simulink model "BLDCMotor"  (R2020a)
settings: Solver=VariableStepAuto  StartTime=0.0  StopTime=10.0  RelTol=1e-3
libraries: simulink x1
settings Model: Creator=Hp  LastModifiedBy=Hp

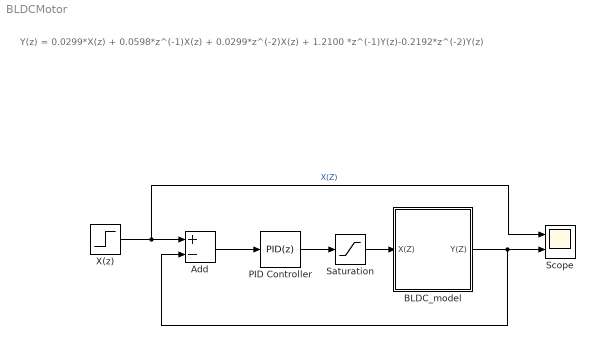
== system BLDCMotor ==
  note: Y(z) = 0.0299*X(z) + 0.0598*z^(-1)X(z) + 0.0299*z^(-2)X(z) + 1.2100 *z^(-1)Y(z)-0.2192*z^(-2)Y(z)
  Add : Sum  Inputs=+-
  BLDC_model : Subsystem
  PID Controller : simulink/Continuous/PID Controller  Controller=PID  Form=Parallel  TimeDomain=Discrete-time  UseExternalTs=off  SampleTime=-1  IntegratorMethod=Forward Euler  FilterMethod=Forward Euler  ControllerParametersSource=internal  P=1.20691388645035  I=59.4220416550733  D=0.00191645853146201  UseFilter=on  N=221.630484004673  TunerSelectOption=Transfer Function Based (PID Tuner App)  InitialConditionSource=internal  InitialConditionForIntegrator=0  InitialConditionForFilter=0  DifferentiatorICPrevScaledInput=0  ExternalReset=none  TrackingMode=off  Kt=1  LimitOutput=off  UpperSaturationLimit=inf  LowerSaturationLimit=-inf  LinearizeAsGain=on  AntiWindupMode=none  Kb=1  POutMin=[]  POutMax=[]  IOutMin=[]  IOutMax=[]  DOutMin=[]  DOutMax=[]  NOutMin=[]  NOutMax=[]  SumOutMin=[]  SumOutMax=[]  SaturationOutMin=[]  SaturationOutMax=[]  PParamMin=[]  PParamMax=[]  IParamMin=[]  IParamMax=[]  DParamMin=[]  DParamMax=[]  NParamMin=[]  NParamMax=[]  KbParamMin=[]  KbParamMax=[]  KtParamMin=[]  KtParamMax=[]  KbOutMin=[]  KbOutMax=[]  KtOutMin=[]  KtOutMax=[]  IntegratorOutMin=[]  IntegratorOutMax=[]  FilterOutMin=[]  FilterOutMax=[]  SumI1OutMin=[]  SumI1OutMax=[]  SumI2OutMin=[]  SumI2OutMax=[]  SumI3OutMin=[]  SumI3OutMax=[]  SumI4OutMin=[]  SumI4OutMax=[]  SumDOutMin=[]  SumDOutMax=[]  DifferentiatorOutMin=[]  DifferentiatorOutMax=[]  FilterDiffOutCoefMin=[]  FilterDiffOutCoefMax=[]  ReciprocalOutMin=[]  ReciprocalOutMax=[]  SumDenOutMin=[]  SumDenOutMax=[]  SumNumOutMin=[]  SumNumOutMax=[]  DivideOutMin=[]  DivideOutMax=[]  UdiffTsProdOutMin=[]  UdiffTsProdOutMax=[]  NTsProdOutMin=[]  NTsProdOutMax=[]  UintegralTsProdOutMin=[]  UintegralTsProdOutMax=[]  UngainTsProdOutMin=[]  UngainTsProdOutMax=[]  IntegratorContinuousStateAttributes=''  IntegratorStateMustResolveToSignalObject=off  IntegratorRTWStateStorageClass=Auto  FilterContinuousStateAttributes=''  FilterStateMustResolveToSignalObject=off  FilterRTWStateStorageClass=Auto  ParallelPVariant=InternalParameters  IdealPVariant=Disabled  IVariant=InternalParameters  DVariant=InternalParameters  IntegratorVariant=Discrete  SatVariant=Disabled  AWVariant=Passthrough  PCopyVariant=Disabled  TRVariant=Disabled  FdbkBlocksVariant=Forward  IdealPFdbkVariant=Disabled  SatFdbkVariant=Disabled  DerivativeFilterVariant=ForwardEulerFilter  NVariant=InternalParameters  NCopyVariant=Disabled  FilterICVariant=InternalICsFilter  IntegratorICVariant=InternalICs  ExternalResetVariant=Disabled  TRSumVariant=Passthrough  SumFdbkVariant=Disabled  SumVariant=Sum_PID  TsampFilterVariant=InternalTs  TsampNgainVariant=Passthrough  TsampIntegralVariant=Passthrough
  Saturation : Saturate  UpperLimit=1  LowerLimit=-1
  Scope : Scope  NumInputPorts=2
  X(z) : Step  SampleTime=0.001
  wires:
  X(z)/1 -> Add/1, Scope/1  "X(Z)"
  BLDC_model/1(Y(Z)) -> Add/2, Scope/2
  PID Controller/1 -> Saturation/1
  Add/1 -> PID Controller/1
  Saturation/1 -> BLDC_model/1(X(Z))

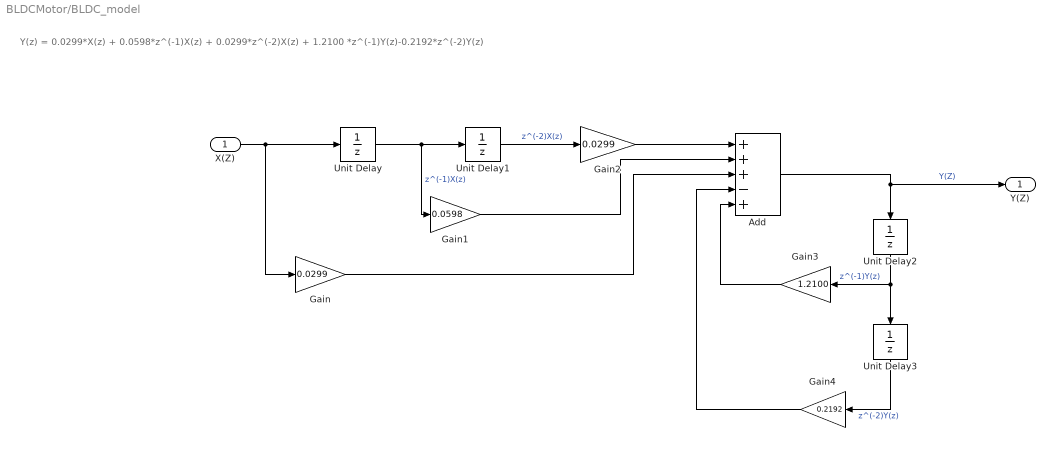
== system BLDCMotor/BLDC_model ==
  note: Y(z) = 0.0299*X(z) + 0.0598*z^(-1)X(z) + 0.0299*z^(-2)X(z) + 1.2100 *z^(-1)Y(z)-0.2192*z^(-2)Y(z)
  X(Z) : Inport
  Add : Sum  Inputs=+++-+
  Gain : Gain  Gain=0.0299
  Gain1 : Gain  Gain=0.0598
  Gain2 : Gain  Gain=0.0299
  Gain3 : Gain  Gain=1.2100
  Gain4 : Gain  Gain=0.2192
  Unit Delay{,1..3} (4 alike) : UnitDelay  SampleTime=-1  HasFrameUpgradeWarning=on
  Y(Z) : Outport
  wires:
  Gain1/1 -> Add/2
  Unit Delay3/1 -> Gain4/1  "z^(-2)Y(z)"
  Unit Delay2/1 -> Gain3/1, Unit Delay3/1  "z^(-1)Y(z)"
  Gain3/1 -> Add/5
  Add/1 -> Y(Z)/1, Unit Delay2/1  "Y(Z)"
  Gain/1 -> Add/3
  Unit Delay1/1 -> Gain2/1  "z^(-2)X(z)"
  Gain4/1 -> Add/4
  Unit Delay/1 -> Gain1/1, Unit Delay1/1  "z^(-1)X(z)"
  Gain2/1 -> Add/1
  X(Z)/1 -> Unit Delay/1, Gain/1
